simulink model "Test2"  (R2025b)
settings: Solver=VariableStepAuto  StartTime=0.0  StopTime=10.0  RelTol=1e-3
settings Model: Creator=henni  LastModifiedBy=henni

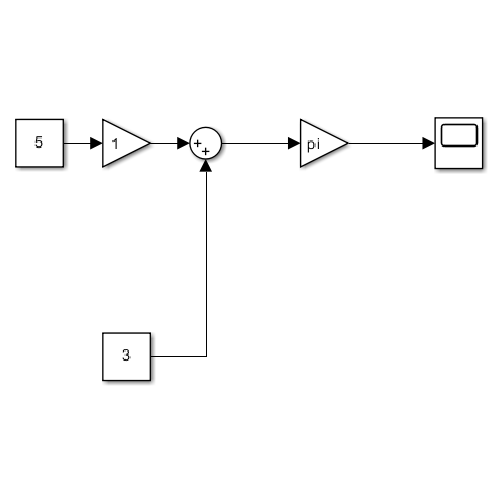
[thumbnail: Simulink's stored preview of the top-level diagram]
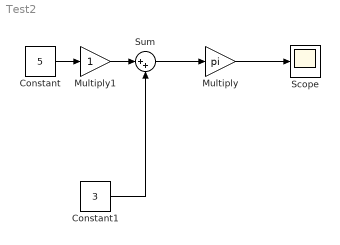
== system Test2 ==
  Constant : Constant  Value=5
  Constant1 : Constant  Value=3
  Multiply : Gain  Gain=pi
  Multiply1 : Gain
  Scope : Scope
      settings: ActiveDisplayYMinimum=15.132741228718345  ActiveDisplayYMaximum=35.132741228718345
  Sum : Sum  Inputs=|++
  wires:
  Constant/1 -> Multiply1/1
  Constant1/1 -> Sum/2
  Multiply/1 -> Scope/1
  Sum/1 -> Multiply/1
  Multiply1/1 -> Sum/1
